simulink model "mcp3208_task"  (Simulink 3.00)
libraries: speclib x1

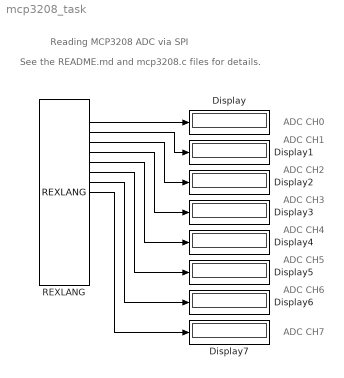
== system mcp3208_task ==
  note: Reading MCP3208 ADC via SPI
  note: See the README.md and mcp3208.c files for details.
  note: ADC CH0
  note: ADC CH1
  note: ADC CH2
  note: ADC CH3
  note: ADC CH4
  note: ADC CH5
  note: ADC CH6
  note: ADC CH7
  Display{,1..7} (8 alike) : Display
      settings: Format=Best fit
  REXLANG : speclib/REXLANG  strs=0  srcname=mcp3208.c  srctype=1: C-like  stack=0  debug=3: Full check  fname=/dev/spidev0.0  p0=/dev/spidev0.0
  wires:
  REXLANG/2 -> Display/1
  REXLANG/3 -> Display1/1
  REXLANG/4 -> Display2/1
  REXLANG/5 -> Display3/1
  REXLANG/6 -> Display4/1
  REXLANG/7 -> Display5/1
  REXLANG/8 -> Display6/1
  REXLANG/9 -> Display7/1
